simulink model "P1"  (R2022a)
settings: Solver=FixedStepAuto  StartTime=0.0  StopTime=10.0  RelTol=1e-3  EnableMultiTasking=on
undefined symbols (not defined in the file): D0, D1, D10, D11, D12, D2, D4, D5, D7, D8, D9, PTA0, PTA2, PTB23, PTB9, PTC16, PTC17, PTC3, PTC4, PTD0, PTD2, PTD3
libraries: frdmk64flib x11
settings Model: ExtModeTrigDuration=5  Creator=ramu7  LastModifiedBy=ramu7
settings OptimizationCC: EnhancedBackFolding=on  PassReuseOutputArgsAs=Individual arguments  ZeroExternalMemoryAtStartup=off  ZeroInternalMemoryAtStartup=off  MaxStackSize=64  OptimizeBlockOrder=speed  DifferentSizesBufferReuse=on  OptimizationCustomize=off  EfficientTunableParamExpr=on
settings DebuggingCC: ParameterTunabilityLossMsg=error
settings HardwareCC: ProdBitPerPointer=32  ProdBitPerSizeT=32  ProdBitPerPtrDiffT=32  ProdLargestAtomicInteger=Long  ProdLargestAtomicFloat=Double  ProdWordSize=32  ProdHWDeviceType=ARM Compatible->ARM Cortex
settings SFSimCC: MATLABDynamicMemAlloc=off
settings RTWCC: SystemTargetFile=ert.tlc  HardwareBoard=NXP FRDM-K64F  TLCOptions="-aInlineSetEventsForThisBaseRateFcn=TLC_FALSE -aSuppressMultiTaskScheduler=TLC_FALSE  -aRateBasedStepFcn=0"  TemplateMakefile=ert_default_tmf  Toolchain=GNU Tools for ARM Embedded Processors
settings CodeAppCC: ForceParamTrailComments=on  IgnoreCustomStorageClasses=off  OperatorAnnotations=on  SimulinkDataObjDesc=on  SFDataObjDesc=on  InsertBlockDesc=on
settings ERTTargetCC: ExtModeTransport=4  ExtModeMexFile=sendToCommService

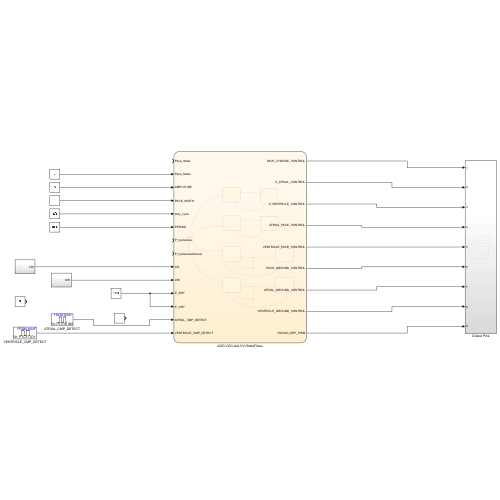
[thumbnail: Simulink's stored preview of the top-level diagram]
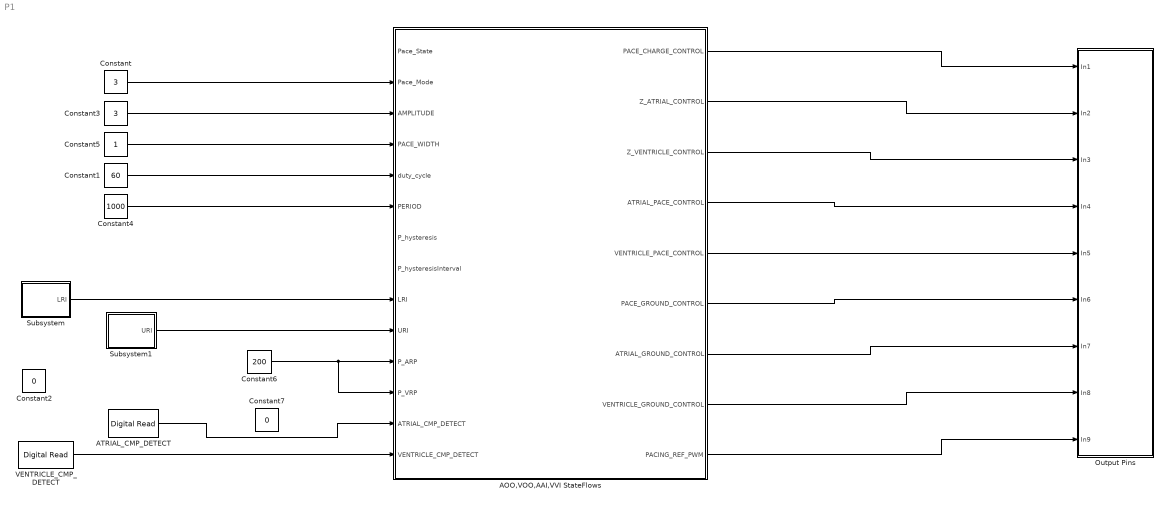
== system P1 ==
  AOO,VOO,AAI,VVI StateFlows : Stateflow chart  TreatAsAtomicUnit=on
      settings: PortSchema="{\"entries\":[{\"content\":{\"sides\":[{\"content\":{\"connectorIds\":[\"In12\",\"In2\",\"In7\",\"In8\",\"In1\",\"In3\",\"In10\",\"In11\",\"In6\",\"In13\",\"In14\",\"In9\",\"In4\",\"In5\"]},\"type\":\"ConnectorPlacement.EquallySpacedRectSide\",\"uuid\":\"9770646f-499d-4715-b3e0-54ec63e9a743\"},{\"content\":{\"connectorIds\":[\"Out1\",\"Out2\",\"Out3\",\"Out4\",\"Out5\",\"Out6\",\"Out7\",\"Out8\",\"Out9\"],\"side\":\"RIGHT\"},\"type\":\"ConnectorPlacement.EquallySpacedRectSide\",\"uuid\":\"05a40026-c63e-4ef0-b71d-820a20f884f3\"},{\"content\":{\"connectorIds\":[],\"side\":\"TOP\"},\"type\":\"ConnectorPlacement.EquallySpacedRectSide\",\"uuid\":\"87d8712c-6353-4ad8-9661-243ca412d6bb\"}]},\"type\":\"ConnectorPlacement.EquallySpacedConnector\",\"uuid\":\"8262e7ac-98b5-44bf-add5-1ad3a0c707a1\"}],\"packageUris\":[\"http://schema.mathworks.com/mf0/Connector/R2020b\"],\"version\":\"1.0\"}"
  ATRIAL_CMP_DETECT : frdmk64flib/Digital Read  Whichpin=PTC16 (D0)  SampleTime=-1
  Constant : Constant  Value=3
  Constant1 : Constant  Value=60
  Constant2 : Constant  Value=0
  Constant3 : Constant  Value=3
  Constant4 : Constant  Value=1000
  Constant5 : Constant
  Constant6 : Constant  Value=200
  Constant7 : Constant  Value=0
  Output Pins : Subsystem
  Subsystem : Subsystem
  Subsystem1 : Subsystem
  VENTRICLE_CMP_DETECT : frdmk64flib/Digital Read  Whichpin=PTC17 (D1)  SampleTime=-1
  wires:
  Constant1/1 -> AOO,VOO,AAI,VVI StateFlows/1(duty_cycle)
  Constant/1 -> AOO,VOO,AAI,VVI StateFlows/2(Pace_Mode)
  VENTRICLE_CMP_DETECT/1 -> AOO,VOO,AAI,VVI StateFlows/5(VENTRICLE_CMP_DETECT)
  Constant3/1 -> AOO,VOO,AAI,VVI StateFlows/7(AMPLITUDE)
  Constant4/1 -> AOO,VOO,AAI,VVI StateFlows/3(PERIOD)
  Constant5/1 -> AOO,VOO,AAI,VVI StateFlows/8(PACE_WIDTH)
  AOO,VOO,AAI,VVI StateFlows/1(PACE_CHARGE_CONTROL) -> Output Pins/1(In1)
  AOO,VOO,AAI,VVI StateFlows/2(Z_ATRIAL_CONTROL) -> Output Pins/2(In2)
  AOO,VOO,AAI,VVI StateFlows/3(Z_VENTRICLE_CONTROL) -> Output Pins/3(In3)
  AOO,VOO,AAI,VVI StateFlows/4(ATRIAL_PACE_CONTROL) -> Output Pins/4(In4)
  AOO,VOO,AAI,VVI StateFlows/5(VENTRICLE_PACE_CONTROL) -> Output Pins/5(In5)
  AOO,VOO,AAI,VVI StateFlows/6(PACE_GROUND_CONTROL) -> Output Pins/6(In6)
  AOO,VOO,AAI,VVI StateFlows/7(ATRIAL_GROUND_CONTROL) -> Output Pins/7(In7)
  AOO,VOO,AAI,VVI StateFlows/8(VENTRICLE_GROUND_CONTROL) -> Output Pins/8(In8)
  AOO,VOO,AAI,VVI StateFlows/9(PACING_REF_PWM) -> Output Pins/9(In9)
  Subsystem/1(LRI) -> AOO,VOO,AAI,VVI StateFlows/6(LRI)
  Subsystem1/1(URI) -> AOO,VOO,AAI,VVI StateFlows/13(URI)
  Constant6/1 -> AOO,VOO,AAI,VVI StateFlows/9(P_VRP), AOO,VOO,AAI,VVI StateFlows/14(P_ARP)
  ATRIAL_CMP_DETECT/1 -> AOO,VOO,AAI,VVI StateFlows/4(ATRIAL_CMP_DETECT)

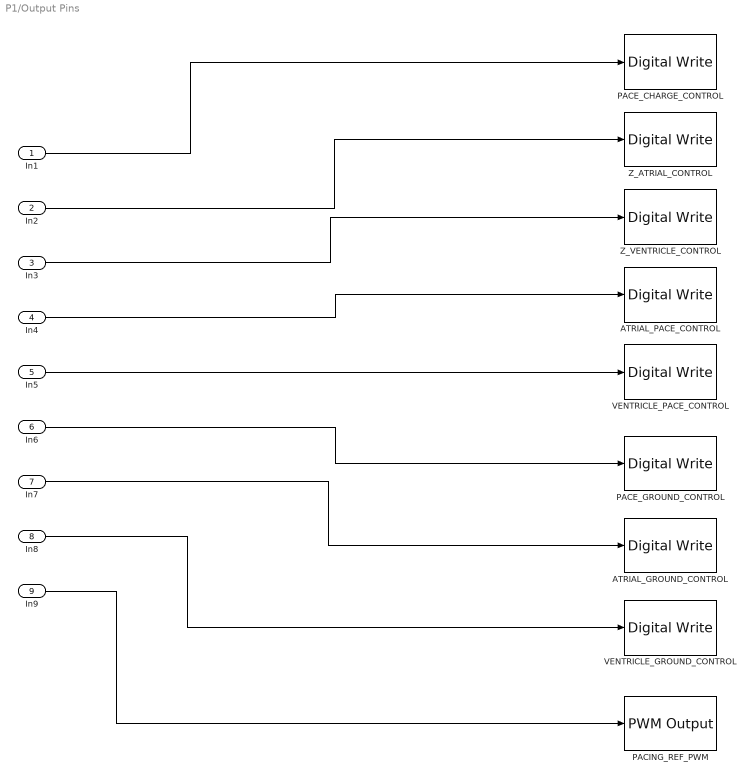
== system P1/Output Pins ==
  In1 : Inport
  In2 : Inport  Port=2
  In3 : Inport  Port=3
  In4 : Inport  Port=4
  In5 : Inport  Port=5
  In6 : Inport  Port=6
  In7 : Inport  Port=7
  In8 : Inport  Port=8
  In9 : Inport  Port=9
  ATRIAL_GROUND_CONTROL : frdmk64flib/Digital Write  Whichpin=PTD2 (D11)
  ATRIAL_PACE_CONTROL : frdmk64flib/Digital Write  Whichpin=PTA0 (D8)
  PACE_CHARGE_CONTROL : frdmk64flib/Digital Write  Whichpin=PTB9 (D2)
  PACE_GROUND_CONTROL : frdmk64flib/Digital Write  Whichpin=PTD0 (D10)
  PACING_REF_PWM : frdmk64flib/PWM Output  Whichpin=PTA2 (D5)  InitialFrequency=2000  InitialDutyCycle=60
  VENTRICLE_GROUND_CONTROL : frdmk64flib/Digital Write  Whichpin=PTD3 (D12)
  VENTRICLE_PACE_CONTROL : frdmk64flib/Digital Write  Whichpin=PTC4 (D9)
  Z_ATRIAL_CONTROL : frdmk64flib/Digital Write  Whichpin=PTB23 (D4)
  Z_VENTRICLE_CONTROL : frdmk64flib/Digital Write  Whichpin=PTC3 (D7)
  wires:
  In2/1 -> Z_ATRIAL_CONTROL/1
  In9/1 -> PACING_REF_PWM/1
  In5/1 -> VENTRICLE_PACE_CONTROL/1
  In7/1 -> ATRIAL_GROUND_CONTROL/1
  In4/1 -> ATRIAL_PACE_CONTROL/1
  In8/1 -> VENTRICLE_GROUND_CONTROL/1
  In6/1 -> PACE_GROUND_CONTROL/1
  In1/1 -> PACE_CHARGE_CONTROL/1
  In3/1 -> Z_VENTRICLE_CONTROL/1

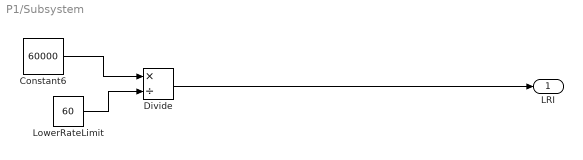
== system P1/Subsystem ==
  Constant6 : Constant  Value=60000
  Divide : Product  Inputs=*/
  LowerRateLimit : Constant  Value=60
  LRI : Outport
  wires:
  Constant6/1 -> Divide/1
  LowerRateLimit/1 -> Divide/2
  Divide/1 -> LRI/1

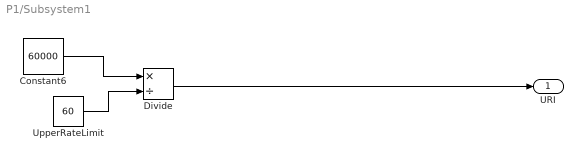
== system P1/Subsystem1 ==
  Constant6 : Constant  Value=60000
  Divide : Product  Inputs=*/
  UpperRateLimit : Constant  Value=60
  URI : Outport
  wires:
  Divide/1 -> URI/1
  UpperRateLimit/1 -> Divide/2
  Constant6/1 -> Divide/1

== stateflow chart P1/AOO,VOO,AAI,VVI StateFlows ==
  state CHARGING_C22_AND_DISCHARGING_C21
    entry:
    ATRIAL_PACE_CONTROL = false
    VENTRICLE_PACE_CONTROL = false
    PACE_CHARGE_CONTROL = true
    PACING_REF_PWM = duty_cycle
    PACE_GROUND_CONTROL = true
    VENTRICLE_PACE_CONTROL = false
    Z_ATRIAL_CONTROL=false
    Z_VENTRICLE_CONTROL=false
    ATRIAL_PACE_CONTROL =false
    ATRIAL_GROUND_CONTROL = true
    VENTRICLE_GROUND_CONTROL=false
  state Atrial_Pacing_by_DISCHARGING_C22
    entry:
    PACE_CHARGE_CONTROL = false
    PACE_GROUND_CONTROL= true
    ATRIAL_PACE_CONTROL =true
    ATRIAL_GROUND_CONTROL = false
    Z_ATRIAL_CONTROL=false
    Z_VENTRICLE_CONTROL=false
    VENTRICLE_GROUND_CONTROL=false
    VENTRICLE_PACE_CONTROL=false
  state CHARGING_C22_AND_DISCHARGING_C21_2
    entry:
    ATRIAL_PACE_CONTROL = false
    VENTRICLE_PACE_CONTROL = false
    PACE_CHARGE_CONTROL = true
    PACING_REF_PWM = duty_cycle
    PACE_GROUND_CONTROL = true
    VENTRICLE_PACE_CONTROL = false
    Z_ATRIAL_CONTROL=false
    Z_VENTRICLE_CONTROL=false
    ATRIAL_PACE_CONTROL =false
    ATRIAL_GROUND_CONTROL = false
    VENTRICLE_GROUND_CONTROL=true
  state Ventricle_Pacing
    entry:
    PACE_CHARGE_CONTROL = false
    PACE_GROUND_CONTROL= true
    ATRIAL_PACE_CONTROL =false
    ATRIAL_GROUND_CONTROL = false
    Z_ATRIAL_CONTROL=false
    Z_VENTRICLE_CONTROL=false
    VENTRICLE_GROUND_CONTROL=false
    VENTRICLE_PACE_CONTROL=true
  state start
  state CHARGING_C22_AND_DISCHARGING_C21_3
    entry:
    ATRIAL_PACE_CONTROL = false
    VENTRICLE_PACE_CONTROL = false
    PACE_CHARGE_CONTROL = true
    PACING_REF_PWM = duty_cycle
    PACE_GROUND_CONTROL = true
    VENTRICLE_PACE_CONTROL = false
    Z_ATRIAL_CONTROL=false
    Z_VENTRICLE_CONTROL=false
    ATRIAL_PACE_CONTROL =false
    ATRIAL_GROUND_CONTROL = true
    VENTRICLE_GROUND_CONTROL=false
  state Atrial_Pacing1
    entry:
    PACE_CHARGE_CONTROL = false
    PACE_GROUND_CONTROL= true
    ATRIAL_PACE_CONTROL =true
    ATRIAL_GROUND_CONTROL = false
    Z_ATRIAL_CONTROL=false
    Z_VENTRICLE_CONTROL=false
    VENTRICLE_GROUND_CONTROL=false
    VENTRICLE_PACE_CONTROL=false
  state CHARGING_C22_AND_DISCHARGING_C21_4
    entry:
    ATRIAL_PACE_CONTROL = false
    VENTRICLE_PACE_CONTROL = false
    PACE_CHARGE_CONTROL = true
    PACING_REF_PWM = duty_cycle
    PACE_GROUND_CONTROL = true
    VENTRICLE_PACE_CONTROL = false
    Z_ATRIAL_CONTROL=false
    Z_VENTRICLE_CONTROL=false
    ATRIAL_PACE_CONTROL =false
    ATRIAL_GROUND_CONTROL = false
    VENTRICLE_GROUND_CONTROL=true
  state Ventricle_Pacing1
    entry:
    PACE_CHARGE_CONTROL = false
    PACE_GROUND_CONTROL= true
    ATRIAL_PACE_CONTROL =false
    ATRIAL_GROUND_CONTROL = false
    Z_ATRIAL_CONTROL=false
    Z_VENTRICLE_CONTROL=false
    VENTRICLE_GROUND_CONTROL=false
    VENTRICLE_PACE_CONTROL=true
  CHARGING_C22_AND_DISCHARGING_C21 -> Atrial_Pacing_by_DISCHARGING_C22 : after(PERIOD - PACE_WIDTH,msec)
  start -> CHARGING_C22_AND_DISCHARGING_C21 [order 1] : [Pace_Mode == 1
      | ]
  Atrial_Pacing_by_DISCHARGING_C22 -> CHARGING_C22_AND_DISCHARGING_C21 : after(PACE_WIDTH,msec)
  CHARGING_C22_AND_DISCHARGING_C21_2 -> Ventricle_Pacing : after(PERIOD - PACE_WIDTH,msec)
  start -> CHARGING_C22_AND_DISCHARGING_C21_2 [order 2] : [Pace_Mode == 2
      | ]
  Ventricle_Pacing -> CHARGING_C22_AND_DISCHARGING_C21_2 : after(PACE_WIDTH,msec)
  (default) -> start
  start -> CHARGING_C22_AND_DISCHARGING_C21_4 [order 4] : [Pace_Mode == 4]
  start -> CHARGING_C22_AND_DISCHARGING_C21_3 [order 3] : [Pace_Mode == 3]
  CHARGING_C22_AND_DISCHARGING_C21_3 -> (junction 103) : after(P_ARP,msec)
  (junction 103) -> Atrial_Pacing1 [order 1] : after(LRI - P_ARP,msec)
  (junction 103) -> (junction 102) [order 2] : [ATRIAL_CMP_DETECT == 1]
  Atrial_Pacing1 -> CHARGING_C22_AND_DISCHARGING_C21_3
  (junction 102) -> CHARGING_C22_AND_DISCHARGING_C21_3
  CHARGING_C22_AND_DISCHARGING_C21_4 -> (junction 100) : after(P_VRP,msec)
  (junction 100) -> Ventricle_Pacing1 [order 1] : after(LRI - P_VRP,msec)
  (junction 100) -> (junction 99) [order 2] : [VENTRICLE_CMP_DETECT == 1]
  Ventricle_Pacing1 -> CHARGING_C22_AND_DISCHARGING_C21_4
  (junction 99) -> CHARGING_C22_AND_DISCHARGING_C21_4
  data: PACE_CHARGE_CONTROL output; Z_ATRIAL_CONTROL output; Z_VENTRICLE_CONTROL output; ATRIAL_PACE_CONTROL output; VENTRICLE_PACE_CONTROL output; PACE_GROUND_CONTROL output; ATRIAL_GROUND_CONTROL output; VENTRICLE_GROUND_CONTROL output; PACING_REF_PWM output; duty_cycle input; Pace_Mode input double; PERIOD input double; ATRIAL_CMP_DETECT input int32; VENTRICLE_CMP_DETECT input boolean; LRI input double; AMPLITUDE input double; PACE_WIDTH input double; P_VRP input double; P_hysteresis input double; P_hysteresisInterval input double; Pace_State input double; URI input double; P_ARP input double
